simulink library "SG_library"  (R2020a)
settings: Solver=VariableStepAuto  StartTime=0.0  StopTime=10.0  RelTol=1e-3
undefined symbols (not defined in the file): a, b, c, IO334, IO397
libraries: speedgoatlib_hdlCoder_IO3xx x54, $bdroot x8, hdlsllib x7, simulink x1, simulink_extras x1
(part 2 of 2)

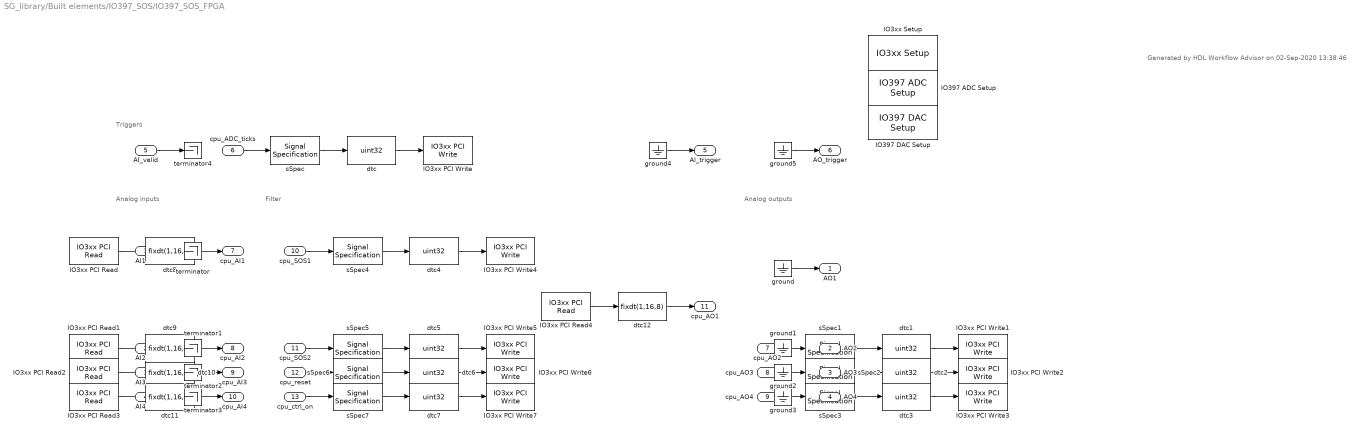
== system SG_library/Built elements/IO397_SOS/IO397_SOS_FPGA ==
  note: Generated by HDL Workflow Advisor on 02-Sep-2020 13:38:46
  note: Triggers
  note: Analog outputs
  note: Filter
  note: Analog inputs
  AI1 : Inport
  AI2 : Inport  Port=2
  AI3 : Inport  Port=3
  AI4 : Inport  Port=4
  AI_valid : Inport  Port=5
  cpu_ADC_ticks : Inport  Port=6
  cpu_AO2 : Inport  Port=7
  cpu_AO3 : Inport  Port=8
  cpu_AO4 : Inport  Port=9
  cpu_SOS1 : Inport  Port=10
  cpu_SOS2 : Inport  Port=11
  cpu_reset : Inport  Port=12
  cpu_ctrl_on : Inport  Port=13
  IO397 ADC Setup : speedgoatlib_hdlCoder_IO3xx/IO397 ADC Setup  module_id=module_id  range1=+-10 V  range2=+-10 V  range3=+-10 V  range4=+-10 V
  IO397 DAC Setup : speedgoatlib_hdlCoder_IO3xx/IO397 DAC Setup  module_id=module_id  span=+-10 V
  IO3xx PCI Read : speedgoatlib_hdlCoder_IO3xx/IO3xx PCI Read  device_id=deviceIdx  module_id=module_id  board_type=IO3xx  port_name=cpu_AI1  port_offset=hex2dec('118')  port_type=uint32  port_dim=1  strobe=0  sample_time=ts
  IO3xx PCI Read1 : speedgoatlib_hdlCoder_IO3xx/IO3xx PCI Read  device_id=deviceIdx  module_id=module_id  board_type=IO3xx  port_name=cpu_AI2  port_offset=hex2dec('11C')  port_type=uint32  port_dim=1  strobe=0  sample_time=ts
  IO3xx PCI Read2 : speedgoatlib_hdlCoder_IO3xx/IO3xx PCI Read  device_id=deviceIdx  module_id=module_id  board_type=IO3xx  port_name=cpu_AI3  port_offset=hex2dec('120')  port_type=uint32  port_dim=1  strobe=0  sample_time=ts
  IO3xx PCI Read3 : speedgoatlib_hdlCoder_IO3xx/IO3xx PCI Read  device_id=deviceIdx  module_id=module_id  board_type=IO3xx  port_name=cpu_AI4  port_offset=hex2dec('124')  port_type=uint32  port_dim=1  strobe=0  sample_time=ts
  IO3xx PCI Read4 : speedgoatlib_hdlCoder_IO3xx/IO3xx PCI Read  device_id=deviceIdx  module_id=module_id  board_type=IO3xx  port_name=cpu_AO1  port_offset=hex2dec('128')  port_type=uint32  port_dim=1  strobe=0  sample_time=ts
  IO3xx PCI Write : speedgoatlib_hdlCoder_IO3xx/IO3xx PCI Write  device_id=deviceIdx  module_id=module_id  board_type=IO3xx  port_name=cpu_ADC_ticks  port_offset=hex2dec('100')  port_type=uint32  port_dim=1  strobe=0  sample_time=ts
  IO3xx PCI Write1 : speedgoatlib_hdlCoder_IO3xx/IO3xx PCI Write  device_id=deviceIdx  module_id=module_id  board_type=IO3xx  port_name=cpu_AO2  port_offset=hex2dec('104')  port_type=uint32  port_dim=1  strobe=0  sample_time=ts
  IO3xx PCI Write2 : speedgoatlib_hdlCoder_IO3xx/IO3xx PCI Write  device_id=deviceIdx  module_id=module_id  board_type=IO3xx  port_name=cpu_AO3  port_offset=hex2dec('108')  port_type=uint32  port_dim=1  strobe=0  sample_time=ts
  IO3xx PCI Write3 : speedgoatlib_hdlCoder_IO3xx/IO3xx PCI Write  device_id=deviceIdx  module_id=module_id  board_type=IO3xx  port_name=cpu_AO4  port_offset=hex2dec('10C')  port_type=uint32  port_dim=1  strobe=0  sample_time=ts
  IO3xx PCI Write4 : speedgoatlib_hdlCoder_IO3xx/IO3xx PCI Write  device_id=deviceIdx  module_id=module_id  board_type=IO3xx  port_name=cpu_SOS1  port_offset=hex2dec('180')  port_type=uint32  port_dim=24  strobe=hex2dec('200')  sample_time=ts
  IO3xx PCI Write5 : speedgoatlib_hdlCoder_IO3xx/IO3xx PCI Write  device_id=deviceIdx  module_id=module_id  board_type=IO3xx  port_name=cpu_SOS2  port_offset=hex2dec('280')  port_type=uint32  port_dim=24  strobe=hex2dec('300')  sample_time=ts
  IO3xx PCI Write6 : speedgoatlib_hdlCoder_IO3xx/IO3xx PCI Write  device_id=deviceIdx  module_id=module_id  board_type=IO3xx  port_name=cpu_reset  port_offset=hex2dec('110')  port_type=uint32  port_dim=1  strobe=0  sample_time=ts
  IO3xx PCI Write7 : speedgoatlib_hdlCoder_IO3xx/IO3xx PCI Write  device_id=deviceIdx  module_id=module_id  board_type=IO3xx  port_name=cpu_ctrl_on  port_offset=hex2dec('114')  port_type=uint32  port_dim=1  strobe=0  sample_time=ts
  IO3xx Setup : speedgoatlib_hdlCoder_IO3xx/IO3xx Setup  mdl_ss_name=IO397_SOS_src/IO397_SOS/IO397_SOS_FPGA  board_type=IO397-50k  fpga_sync_mode=on  reset_mode=on  device_id=deviceIdx  module_id=module_id  pci_slot=slot  fpga_mat_file=C:\Speedgoat\Build\IO397_SOS\hdlsrc\IO397_SOS_src\IO397_SOS_FPGA.mat  timestamp_mcs=09/02/20 13:37:55  timestamp=2009021330  tsreg=hex2dec('8')  bsf_file=IO397_SOS_FPGA_2009021330.mcs  mcs=0
  dtc{,1..7} (8 alike) : DataTypeConversion  OutDataTypeStr=uint32  ConvertRealWorld=Stored Integer (SI)  RndMeth=Zero
  dtc{8..12} (5 alike) : DataTypeConversion  OutDataTypeStr=fixdt(1,16,8)  ConvertRealWorld=Stored Integer (SI)  RndMeth=Zero
  ground{,1..5} (6 alike) : Ground
  sSpec : SignalSpecification  OutDataTypeStr=fixdt(0,32,0)
  sSpec1 : SignalSpecification  OutDataTypeStr=fixdt(1,16,8)
  sSpec2 : SignalSpecification  OutDataTypeStr=fixdt(1,16,8)
  sSpec3 : SignalSpecification  OutDataTypeStr=fixdt(1,16,8)
  sSpec4 : SignalSpecification  OutDataTypeStr=fixdt(1,32,20)
  sSpec5 : SignalSpecification  OutDataTypeStr=fixdt(1,32,20)
  sSpec6 : SignalSpecification  OutDataTypeStr=fixdt('boolean')
  sSpec7 : SignalSpecification  OutDataTypeStr=fixdt('boolean')
  terminator{,1..4} (5 alike) : Terminator
  AO1 : Outport  VectorParamsAs1DForOutWhenUnconnected=off
  AO2 : Outport  Port=2  VectorParamsAs1DForOutWhenUnconnected=off
  AO3 : Outport  Port=3  VectorParamsAs1DForOutWhenUnconnected=off
  AO4 : Outport  Port=4  VectorParamsAs1DForOutWhenUnconnected=off
  AI_trigger : Outport  Port=5  VectorParamsAs1DForOutWhenUnconnected=off
  AO_trigger : Outport  Port=6  VectorParamsAs1DForOutWhenUnconnected=off
  cpu_AI1 : Outport  Port=7  VectorParamsAs1DForOutWhenUnconnected=off
  cpu_AI2 : Outport  Port=8  VectorParamsAs1DForOutWhenUnconnected=off
  cpu_AI3 : Outport  Port=9  VectorParamsAs1DForOutWhenUnconnected=off
  cpu_AI4 : Outport  Port=10  VectorParamsAs1DForOutWhenUnconnected=off
  cpu_AO1 : Outport  Port=11  VectorParamsAs1DForOutWhenUnconnected=off
  wires:
  IO3xx PCI Read4/1 -> dtc12/1
  dtc12/1 -> cpu_AO1/1
  IO3xx PCI Read3/1 -> dtc11/1
  dtc11/1 -> cpu_AI4/1
  IO3xx PCI Read2/1 -> dtc10/1
  dtc10/1 -> cpu_AI3/1
  IO3xx PCI Read1/1 -> dtc9/1
  dtc9/1 -> cpu_AI2/1
  IO3xx PCI Read/1 -> dtc8/1
  dtc8/1 -> cpu_AI1/1
  ground5/1 -> AO_trigger/1
  ground4/1 -> AI_trigger/1
  ground3/1 -> AO4/1
  ground2/1 -> AO3/1
  ground1/1 -> AO2/1
  ground/1 -> AO1/1
  dtc7/1 -> IO3xx PCI Write7/1
  sSpec7/1 -> dtc7/1
  cpu_ctrl_on/1 -> sSpec7/1
  dtc6/1 -> IO3xx PCI Write6/1
  sSpec6/1 -> dtc6/1
  cpu_reset/1 -> sSpec6/1
  dtc5/1 -> IO3xx PCI Write5/1
  sSpec5/1 -> dtc5/1
  cpu_SOS2/1 -> sSpec5/1
  dtc4/1 -> IO3xx PCI Write4/1
  sSpec4/1 -> dtc4/1
  cpu_SOS1/1 -> sSpec4/1
  dtc3/1 -> IO3xx PCI Write3/1
  sSpec3/1 -> dtc3/1
  cpu_AO4/1 -> sSpec3/1
  dtc2/1 -> IO3xx PCI Write2/1
  sSpec2/1 -> dtc2/1
  cpu_AO3/1 -> sSpec2/1
  dtc1/1 -> IO3xx PCI Write1/1
  sSpec1/1 -> dtc1/1
  cpu_AO2/1 -> sSpec1/1
  dtc/1 -> IO3xx PCI Write/1
  sSpec/1 -> dtc/1
  cpu_ADC_ticks/1 -> sSpec/1
  AI_valid/1 -> terminator4/1
  AI4/1 -> terminator3/1
  AI3/1 -> terminator2/1
  AI2/1 -> terminator1/1
  AI1/1 -> terminator/1

== matlab function SG_library/Source elements/Get ADC ticks/MATLAB Function ==
  data: f_adc input; f_fpga input; ticks output; os input
function ticks = fcn(f_adc, f_fpga, os)
    ticks = uint32(f_fpga/(f_adc*os) - 1);
end
